simulink model "six_dof_simulation"  (R2020a)
settings: Solver=ode15s  StartTime=0.0  StopTime=1000  FixedStep=0.02  RelTol=1e-3
values from neighbouring files (symbols this model uses):
  u1max = 25*pi/180    (= 0.436332312999)    [initialise.m]
  u1min = -25*pi/180    (= -0.436332312999)    [initialise.m]
  u2max = 10*pi/180    (= 0.174532925199)    [initialise.m]
  u2min = -25*pi/180    (= -0.436332312999)    [initialise.m]
  u3max = 30*pi/180    (= 0.523598775598)    [initialise.m]
  u3min = -30*pi/180    (= -0.523598775598)    [initialise.m]
  u4max = 10*pi/180    (= 0.174532925199)    [initialise.m]
  u4min = 0    [initialise.m]
  u5max = 10*pi/180    (= 0.174532925199)    [initialise.m]
  u5min = 0    [initialise.m]
  x0 = [85 ... (first row only)    [initialise.m]
undefined symbols (not defined in the file or in its folder): RB211, RCAM_plant
libraries: simulink_extras x3, aerolibutil x2, aerolibfltsims x2, aerolibanimutils x1, vrlib x1
settings Model: Creator=Khojasteh Mirza  LastModifiedBy=Khojasteh Mirza
settings SolverCC: InitialStep=0.01
settings DataIOCC: ReturnWorkspaceOutputs=off

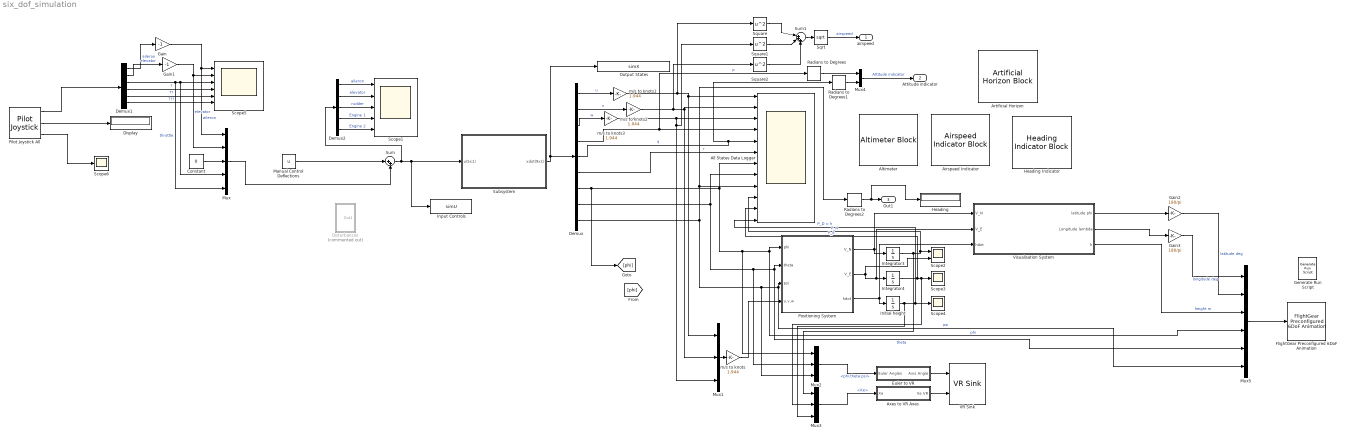
== system six_dof_simulation ==
  Airspeed Indicator : AirspeedIndicatorBlock  ScaleMax=350
  All States Data Logger : Scope  NumInputPorts=12
  Altimeter : AltimeterBlock
  Artificial Horizon : ArtificialHorizonBlock
  Axes to VR Axes : Subsystem
  Constant : Constant  Value=0
  Demux : Demux  Outputs=9
  Demux1 : Demux  Outputs=6
  Demux2 : Demux  Outputs=5
  Display : Display
  Disturbances : Subsystem  Commented=on
  Euler to VR : Subsystem
  FlightGear Preconfigured 6DoF Animation : aerolibfltsims/FlightGear Preconfigured 6DoF Animation  xFlightGearVersion=v2018.1  DestinationIpAddress=127.0.0.1  DestinationPort=5502  SampleTime=1/30  packetVersion=24
  Gain : Gain  Gain=-1
  Gain1 : Gain  Gain=-1
  Gain2 : Gain  Gain=180/pi
  Gain3 : Gain  Gain=180/pi
  Generate Run Script : aerolibfltsims/Generate Run Script  Architecture=Win64  dataFlow=Send  GeometryModelName=757-200-RB211  AirportId=PHNL  RunwayId=26L  InitialAltitude=1000  InitialHeading=260  OffsetDistance=0  OffsetAzimuth=0  InstallScenery=off  DisableShaders=on  OriginAddress=127.0.0.1  DestinationPort=5502  OriginPort=5505  LocalAddress=127.0.0.1  OutputFileName=runfg.bat  FlightGearBaseDirectory=D:\FlightGear 2018.1.1
  Heading : Display
  Heading Indicator : HeadingIndicatorBlock
  Initial height : Integrator  InitialCondition=1000
  Input Controls : ToWorkspace  VariableName=simU  SaveFormat=Timeseries  SampleTime=-1
  Integrator3 : Integrator
  Integrator4 : Integrator
  Manual Control Deflections : Constant  Value=u
  Mux : Mux  Inputs=5
  Mux1 : Mux  Inputs=3
  Mux2 : Mux  Inputs=3
  Mux3 : Mux  Inputs=3
  Mux4 : Mux  Inputs=2
  Mux5 : Mux  Inputs=6
  Output States : ToWorkspace  VariableName=simX  SaveFormat=Timeseries  SampleTime=-1
  Pilot Joystick All : aerolibanimutils/Pilot Joystick  JoystickID=Joystick1  OutputConfiguration=AllOutputs  SampleTime=1/50
  Positioning System : Subsystem
  Radians to Degrees : simulink_extras/Transformations/Radians to Degrees
  Radians to Degrees1 : simulink_extras/Transformations/Radians to Degrees
  Radians to Degrees2 : simulink_extras/Transformations/Radians to Degrees
  Scope1 : Scope  NumInputPorts=5
  Scope2 : Scope  NumInputPorts=2
  Scope3 : Scope
  Scope4 : Scope
  Scope5 : Scope  NumInputPorts=6
  Scope6 : Scope
  Sqrt : Sqrt  SaturateOnIntegerOverflow=on
  Square : Math  Operator=square  SaturateOnIntegerOverflow=on
  Square1 : Math  Operator=square  SaturateOnIntegerOverflow=on
  Square2 : Math  Operator=square  SaturateOnIntegerOverflow=on
  Subsystem : Subsystem
  Sum : Sum  Inputs=|++
  Sum1 : Sum  Inputs=|+++
  VR Sink : vrlib/VR Sink  InstantiateOnLoad=on  SampleTime=0.1  ViewEnable=on  RemoteChange=off  RemoteView=off  FieldsWritten=HL20.rotation.4.1.1.double#HL20.translation.3.1.1.double  WorldFileName=aeroblk_HL20.wrl  WorldDescription=aeroblk_HL20  AutoView=on  VideoDimensions=[]  AllowVariableSize=off
  Visualisation System : Subsystem
  m/s to knots{,1..3} (4 alike) : Gain  Gain=1.944
  airspeed : Outport
  Attitude indicator : Outport  Port=2
  Out1 : Outport  Port=3
  wires:
  Manual Control Deflections/1 -> Sum/1
  Sum/1 -> Demux2/1, Input Controls/1, Subsystem/1(u(5x1))
  Subsystem/1(xdot(9x1)) -> Demux/1, Output States/1
  Demux/4 -> Radians to Degrees/1, All States Data Logger/4  "p"
  Demux/3 -> m/s to knots3/1  "w"
  Demux/2 -> m/s to knots2/1  "v"
  Demux/1 -> m/s to knots1/1  "u"
  Demux/7 -> [phi], All States Data Logger/7, Mux2/1, Mux5/4, Positioning System/1(phi)  "phi"
  Demux/8 -> All States Data Logger/8, Mux2/2, Mux5/5, Positioning System/2(theta)  "theta"
  Demux/9 -> All States Data Logger/9, Radians to Degrees2/1, Mux2/3, Mux5/6, Positioning System/3(psi)  "psi"
  Demux2/1 -> Scope1/1  "aileron"
  Demux2/2 -> Scope1/2  "elevator"
  Demux2/3 -> Scope1/3  "rudder"
  Demux2/4 -> Scope1/4  "Engine 1"
  Demux2/5 -> Scope1/5  "Engine 2"
  Demux/6 -> All States Data Logger/6  "r"
  Positioning System/1(V_N) -> Integrator3/1, Visualisation System/1(V_N)
  Integrator3/1 -> Mux3/1, All States Data Logger/10, Scope2/1  "P_N"
  Positioning System/2(V_E) -> Visualisation System/2(V_E), Integrator4/1, Scope2/2
  Integrator4/1 -> All States Data Logger/11, Mux3/2, Scope3/1  "P_E"
  Initial height/1 -> Mux3/3, All States Data Logger/12, Scope4/1  "P_D = h"
  Positioning System/3(hdot) -> Initial height/1, Visualisation System/3(hdot)
  Axes to VR Axes/1(Xe VR) -> VR Sink/2
  Euler to VR/1(Axis Angle) -> VR Sink/1
  Mux3/1 -> Axes to VR Axes/1(Xe)  "<Xe>"
  Mux2/1 -> Euler to VR/1(Euler Angles)  "<phi;theta;psi>"
  Demux1/4 -> Scope5/4  "?"
  Demux1/1 -> Gain/1  "aileron"
  Demux1/6 -> Scope5/6  "???"
  Pilot Joystick All/1 -> Demux1/1
  Demux1/5 -> Scope5/5  "??"
  Pilot Joystick All/2 -> Display/1
  Demux1/3 -> Mux/5, Scope5/3, Mux/4  "throttle"
  Demux1/2 -> Gain1/1  "elevator"
  Pilot Joystick All/3 -> Scope6/1
  Constant/1 -> Mux/3
  Square/1 -> Sum1/1
  Square1/1 -> Sum1/2
  Square2/1 -> Sum1/3
  Sum1/1 -> Sqrt/1
  Sqrt/1 -> airspeed/1  "airspeed"
  Mux4/1 -> Attitude indicator/1  "Attitude indicator"
  Radians to Degrees/1 -> Mux4/1
  Radians to Degrees1/1 -> Mux4/2
  Radians to Degrees2/1 -> Heading/1, Out1/1
  Gain/1 -> Mux/1, Scope5/1  "aileron"
  Gain1/1 -> Mux/2, Scope5/2  "elevator"
  Mux5/1 -> FlightGear Preconfigured 6DoF Animation/1
  Mux/1 -> Sum/2
  Gain3/1 -> Mux5/1  "longitude deg"
  Gain2/1 -> Mux5/2  "latitude deg"
  Visualisation System/3(h) -> Mux5/3  "height m"
  Visualisation System/1(latitude phi) -> Gain2/1
  Visualisation System/2(Longitude lambda) -> Gain3/1
  Mux1/1 -> m/s to knots/1
  m/s to knots/1 -> Positioning System/4(u,v,w)
  Demux/5 -> All States Data Logger/5, Radians to Degrees1/1  "q"
  m/s to knots1/1 -> Square/1, Mux1/1, All States Data Logger/1
  m/s to knots2/1 -> Square2/1, Mux1/2, All States Data Logger/2
  m/s to knots3/1 -> Square1/1, Mux1/3, All States Data Logger/3

== system six_dof_simulation/Axes to VR Axes ==
  Xe : Inport
  Concatenate : Concatenate  NumInputs=3
  Demux : Demux  Outputs=3
      settings: DisplayOption=none
  rad-->deg : Gain  Gain=-1  SaturateOnIntegerOverflow=on  OutDataTypeStr=Inherit: Same as input  ParamDataTypeStr=Inherit: Same as input
  rad-->deg1 : Gain  Gain=-1  SaturateOnIntegerOverflow=on  OutDataTypeStr=Inherit: Same as input  ParamDataTypeStr=Inherit: Same as input
  Xe VR : Outport  VectorParamsAs1DForOutWhenUnconnected=off
  wires:
  Xe/1 -> Demux/1
  Demux/1 -> Concatenate/1
  Demux/2 -> rad-->deg/1
  Demux/3 -> rad-->deg1/1
  Concatenate/1 -> Xe VR/1
  rad-->deg1/1 -> Concatenate/2
  rad-->deg/1 -> Concatenate/3

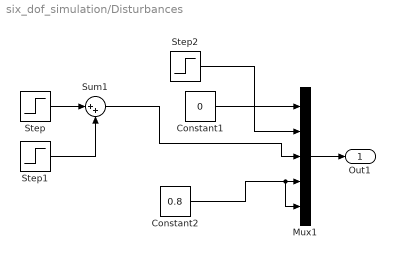
== system six_dof_simulation/Disturbances ==
  Constant1 : Constant  Value=0
  Constant2 : Constant  Value=0.8
  Mux1 : Mux  Inputs=5
  Step : Step  Time=10  After=-25*(pi/180)  SampleTime=0
  Step1 : Step  Time=60  After=10*(pi/180)  SampleTime=0
  Step2 : Step  Time=5  After=-10*(pi/180)  SampleTime=0
  Sum1 : Sum  Inputs=|++
  Out1 : Outport
  wires:
  Mux1/1 -> Out1/1
  Step/1 -> Sum1/1
  Step1/1 -> Sum1/2
  Constant1/1 -> Mux1/1
  Sum1/1 -> Mux1/3
  Step2/1 -> Mux1/2
  Constant2/1 -> Mux1/5, Mux1/4

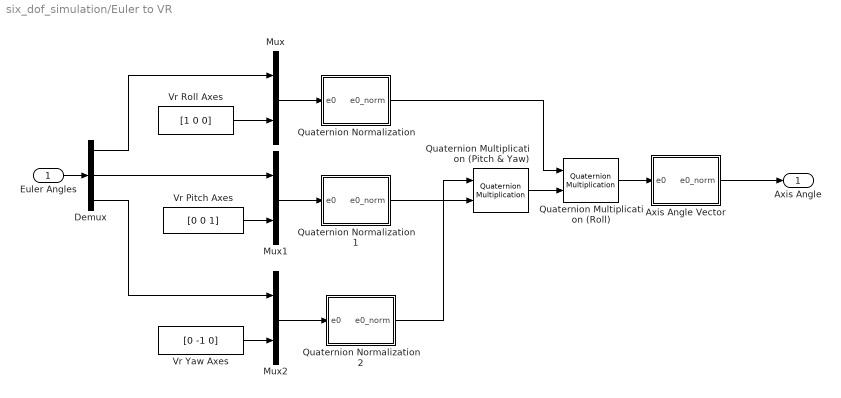
== system six_dof_simulation/Euler to VR ==
  Euler Angles : Inport
  Axis Angle Vector : Subsystem
  Demux : Demux  Outputs=3
      settings: DisplayOption=none
  Mux : Mux  Inputs=2
  Mux1 : Mux  Inputs=2
  Mux2 : Mux  Inputs=2
  Quaternion Multiplication (Pitch & Yaw) : aerolibutil/Quaternion Multiplication
  Quaternion Multiplication (Roll) : aerolibutil/Quaternion Multiplication
  Quaternion Normalization : Subsystem
  Quaternion Normalization1 : Subsystem
  Quaternion Normalization2 : Subsystem
  Vr Pitch Axes : Constant  Value=[0 0 1]
  Vr Roll Axes : Constant  Value=[1 0 0]
  Vr Yaw Axes : Constant  Value=[0 -1 0]
  Axis Angle : Outport  VectorParamsAs1DForOutWhenUnconnected=off
  wires:
  Quaternion Multiplication (Roll)/1 -> Axis Angle Vector/1(e0)
  Quaternion Multiplication (Pitch & Yaw)/1 -> Quaternion Multiplication (Roll)/2
  Axis Angle Vector/1(e0_norm) -> Axis Angle/1
  Quaternion Normalization/1(e0_norm) -> Quaternion Multiplication (Roll)/1
  Quaternion Normalization2/1(e0_norm) -> Quaternion Multiplication (Pitch & Yaw)/1
  Quaternion Normalization1/1(e0_norm) -> Quaternion Multiplication (Pitch & Yaw)/2
  Mux2/1 -> Quaternion Normalization2/1(e0)
  Mux1/1 -> Quaternion Normalization1/1(e0)
  Mux/1 -> Quaternion Normalization/1(e0)
  Demux/3 -> Mux2/1
  Vr Yaw Axes/1 -> Mux2/2
  Demux/2 -> Mux1/1
  Vr Pitch Axes/1 -> Mux1/2
  Demux/1 -> Mux/1
  Vr Roll Axes/1 -> Mux/2
  Euler Angles/1 -> Demux/1

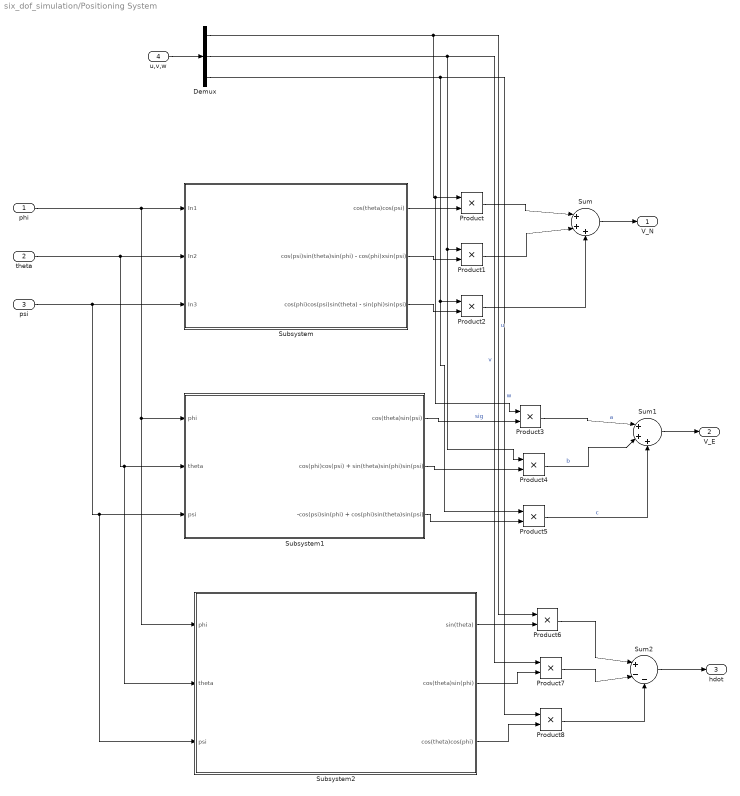
== system six_dof_simulation/Positioning System ==
  phi : Inport
  theta : Inport  Port=2
  psi : Inport  Port=3
  u,v,w : Inport  Port=4
  Demux : Demux  Outputs=3
  Product{,1..8} (9 alike) : Product
  Subsystem : Subsystem
  Subsystem1 : Subsystem
  Subsystem2 : Subsystem
  Sum : Sum  Inputs=|+++
  Sum1 : Sum  Inputs=|+++
  Sum2 : Sum  Inputs=|+--
  V_N : Outport
  V_E : Outport  Port=2
  hdot : Outport  Port=3
  wires:
  u,v,w/1 -> Demux/1
  Demux/1 -> Product6/1, Product3/1, Product/1  "u"
  Demux/2 -> Product7/1, Product4/1, Product1/1  "v"
  Demux/3 -> Product8/1, Product5/1, Product2/1  "w"
  phi/1 -> Subsystem2/1(phi), Subsystem1/1(phi), Subsystem/1(In1)
  psi/1 -> Subsystem/3(In3), Subsystem2/3(psi), Subsystem1/3(psi)
  Subsystem/1(cos(theta)cos(psi)) -> Product/2
  Product/1 -> Sum/1
  Subsystem/2(cos(psi)sin(theta)sin(phi) - cos(phi)xsin(psi)) -> Product1/2
  Product1/1 -> Sum/2
  Subsystem/3(cos(phi)cos(psi)sin(theta) - sin(phi)sin(psi)) -> Product2/2
  Product2/1 -> Sum/3
  Sum/1 -> V_N/1
  theta/1 -> Subsystem2/2(theta), Subsystem1/2(theta), Subsystem/2(In2)
  Sum1/1 -> V_E/1
  Product5/1 -> Sum1/3  "c"
  Product4/1 -> Sum1/2  "b"
  Product3/1 -> Sum1/1  "a"
  Subsystem1/1(cos(theta)sin(psi)) -> Product3/2  "sig"
  Subsystem1/2(cos(phi)cos(psi) + sin(theta)sin(phi)sin(psi)) -> Product4/2
  Subsystem1/3(-cos(psi)sin(phi) + cos(phi)sin(theta)sin(psi)) -> Product5/2
  Subsystem2/1(sin(theta)) -> Product6/2
  Subsystem2/2(cos(theta)sin(phi)) -> Product7/2
  Subsystem2/3(cos(theta)cos(phi)) -> Product8/2
  Product6/1 -> Sum2/1
  Product7/1 -> Sum2/2
  Product8/1 -> Sum2/3
  Sum2/1 -> hdot/1

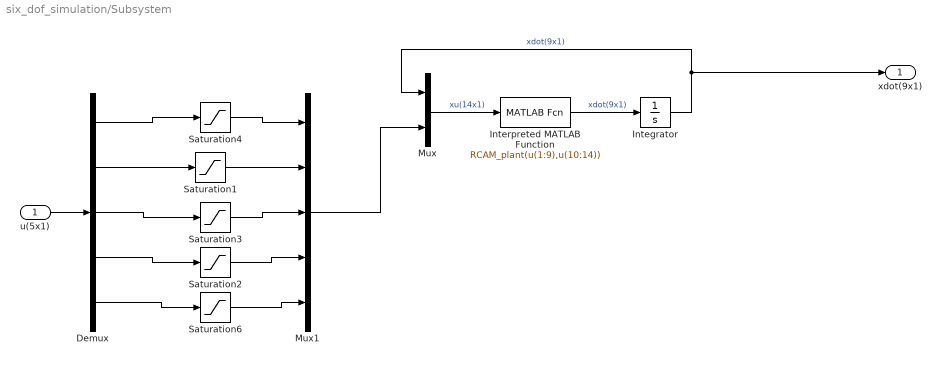
== system six_dof_simulation/Subsystem ==
  u(5x1) : Inport
  Demux : Demux  Outputs=5
  Integrator : Integrator  InitialCondition=x0
  Interpreted MATLAB Function : MATLABFcn  MATLABFcn=RCAM_plant(u(1:9),u(10:14))
  Mux : Mux  Inputs=2
  Mux1 : Mux  Inputs=5
  Saturation1 : Saturate  UpperLimit=u2max  LowerLimit=u2min
  Saturation2 : Saturate  UpperLimit=u4max  LowerLimit=u4min
  Saturation3 : Saturate  UpperLimit=u3max  LowerLimit=u3min
  Saturation4 : Saturate  UpperLimit=u1max  LowerLimit=u1min
  Saturation6 : Saturate  UpperLimit=u5max  LowerLimit=u5min
  xdot(9x1) : Outport
  wires:
  Interpreted MATLAB Function/1 -> Integrator/1  "xdot(9x1)"
  Integrator/1 -> xdot(9x1)/1, Mux/1  "xdot(9x1)"
  Mux/1 -> Interpreted MATLAB Function/1  "xu(14x1)"
  Demux/1 -> Saturation4/1
  Demux/2 -> Saturation1/1
  Demux/3 -> Saturation3/1
  Demux/4 -> Saturation2/1
  Demux/5 -> Saturation6/1
  Saturation4/1 -> Mux1/1
  Saturation1/1 -> Mux1/2
  Saturation3/1 -> Mux1/3
  Saturation2/1 -> Mux1/4
  Saturation6/1 -> Mux1/5
  u(5x1)/1 -> Demux/1
  Mux1/1 -> Mux/2

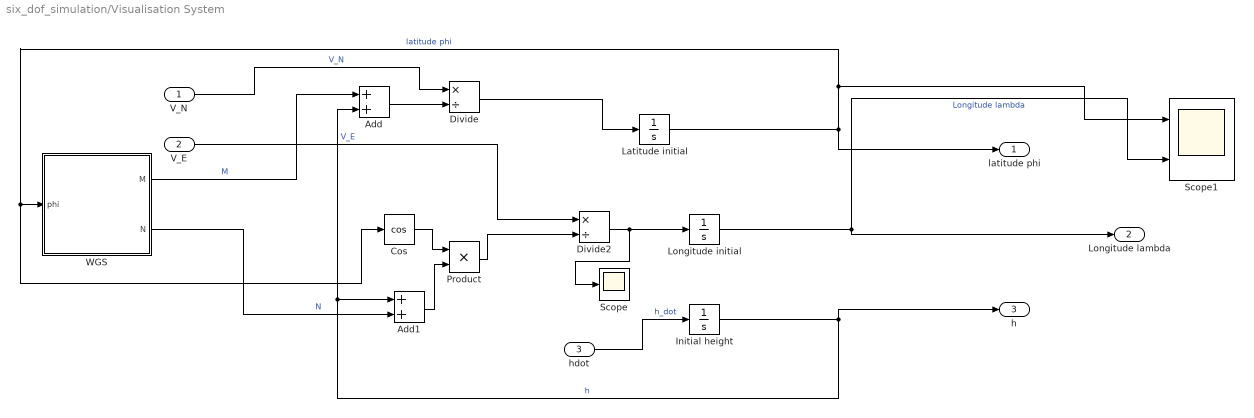
== system six_dof_simulation/Visualisation System ==
  V_N : Inport
  V_E : Inport  Port=2
  hdot : Inport  Port=3
  Add : Sum
  Add1 : Sum
  Cos : Trigonometry  Operator=cos  ApproximationMethod=CORDIC
  Divide : Product  Inputs=*/
  Divide2 : Product  Inputs=*/
  Initial height : Integrator  InitialCondition=1000
  "Latitude initial " : Integrator  InitialCondition=deg2rad(21.32451389)
  Longitude initial : Integrator  InitialCondition=deg2rad(-157.92507222)
  Product : Product
  Scope : Scope
  Scope1 : Scope  NumInputPorts=2
  WGS : Subsystem
  latitude phi : Outport
  Longitude lambda : Outport  Port=2
  h : Outport  Port=3
  wires:
  V_N/1 -> Divide/1  "V_N"
  V_E/1 -> Divide2/1  "V_E"
  WGS/1(M) -> Add/1  "M"
  WGS/2(N) -> Add1/2  "N"
  "Latitude initial "/1 -> latitude phi/1, Cos/1, WGS/1(phi), Scope1/1  "latitude phi"
  Divide/1 -> "Latitude initial "/1
  Initial height/1 -> h/1, Add1/1, Add/2  "h"
  hdot/1 -> Initial height/1  "h_dot"
  Add/1 -> Divide/2
  Longitude initial/1 -> Longitude lambda/1, Scope1/2  "Longitude lambda"
  Add1/1 -> Product/2
  Cos/1 -> Product/1
  Divide2/1 -> Longitude initial/1, Scope/1
  Product/1 -> Divide2/2

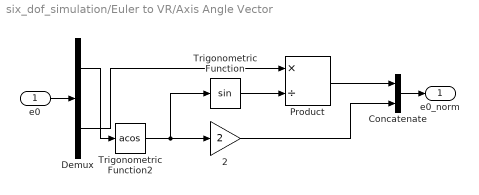
== system six_dof_simulation/Euler to VR/Axis Angle Vector ==
  e0 : Inport
  2 : Gain  Gain=2  SaturateOnIntegerOverflow=on  OutDataTypeStr=Inherit: Same as input  ParamDataTypeStr=Inherit: Same as input
  Concatenate : Concatenate
  Demux : Demux  Outputs=[1 3 ]
      settings: DisplayOption=none
  Product : Product  Inputs=*/  InputSameDT=on  SaturateOnIntegerOverflow=on  OutDataTypeStr=Inherit: Same as first input
  Trigonometric Function : Trigonometry
  Trigonometric Function2 : Trigonometry  Operator=acos
  e0_norm : Outport  VectorParamsAs1DForOutWhenUnconnected=off
  wires:
  Demux/1 -> Trigonometric Function2/1
  Demux/2 -> Product/1
  Concatenate/1 -> e0_norm/1
  Product/1 -> Concatenate/1
  2/1 -> Concatenate/2
  Trigonometric Function/1 -> Product/2
  Trigonometric Function2/1 -> Trigonometric Function/1, 2/1
  e0/1 -> Demux/1

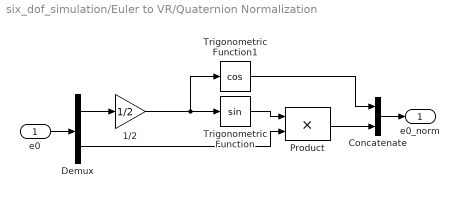
== system six_dof_simulation/Euler to VR/Quaternion Normalization ==
  e0 : Inport
  1/2 : Gain  Gain=1/2  SaturateOnIntegerOverflow=on  OutDataTypeStr=Inherit: Same as input  ParamDataTypeStr=Inherit: Same as input
  Concatenate : Concatenate
  Demux : Demux  Outputs=[1 3]
      settings: DisplayOption=none
  Product : Product  InputSameDT=on  SaturateOnIntegerOverflow=on  OutDataTypeStr=Inherit: Same as first input
  Trigonometric Function : Trigonometry
  Trigonometric Function1 : Trigonometry  Operator=cos
  e0_norm : Outport  VectorParamsAs1DForOutWhenUnconnected=off
  wires:
  Trigonometric Function1/1 -> Concatenate/1
  Demux/2 -> Product/2
  Demux/1 -> 1/2/1
  Concatenate/1 -> e0_norm/1
  Product/1 -> Concatenate/2
  Trigonometric Function/1 -> Product/1
  1/2/1 -> Trigonometric Function1/1, Trigonometric Function/1
  e0/1 -> Demux/1

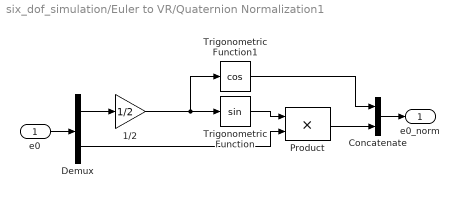
== system six_dof_simulation/Euler to VR/Quaternion Normalization1 ==
  e0 : Inport
  1/2 : Gain  Gain=1/2  SaturateOnIntegerOverflow=on  OutDataTypeStr=Inherit: Same as input  ParamDataTypeStr=Inherit: Same as input
  Concatenate : Concatenate
  Demux : Demux  Outputs=[1 3]
      settings: DisplayOption=none
  Product : Product  InputSameDT=on  SaturateOnIntegerOverflow=on  OutDataTypeStr=Inherit: Same as first input
  Trigonometric Function : Trigonometry
  Trigonometric Function1 : Trigonometry  Operator=cos
  e0_norm : Outport  VectorParamsAs1DForOutWhenUnconnected=off
  wires:
  e0/1 -> Demux/1
  1/2/1 -> Trigonometric Function/1, Trigonometric Function1/1
  Trigonometric Function/1 -> Product/1
  Product/1 -> Concatenate/2
  Concatenate/1 -> e0_norm/1
  Demux/1 -> 1/2/1
  Demux/2 -> Product/2
  Trigonometric Function1/1 -> Concatenate/1

== system six_dof_simulation/Euler to VR/Quaternion Normalization2 ==
  e0 : Inport
  1/2 : Gain  Gain=1/2  SaturateOnIntegerOverflow=on  OutDataTypeStr=Inherit: Same as input  ParamDataTypeStr=Inherit: Same as input
  Concatenate : Concatenate
  Demux : Demux  Outputs=[1 3]
      settings: DisplayOption=none
  Product : Product  InputSameDT=on  SaturateOnIntegerOverflow=on  OutDataTypeStr=Inherit: Same as first input
  Trigonometric Function : Trigonometry
  Trigonometric Function1 : Trigonometry  Operator=cos
  e0_norm : Outport  VectorParamsAs1DForOutWhenUnconnected=off
  wires:
  Trigonometric Function1/1 -> Concatenate/1
  Demux/2 -> Product/2
  Demux/1 -> 1/2/1
  Concatenate/1 -> e0_norm/1
  Product/1 -> Concatenate/2
  Trigonometric Function/1 -> Product/1
  1/2/1 -> Trigonometric Function1/1, Trigonometric Function/1
  e0/1 -> Demux/1

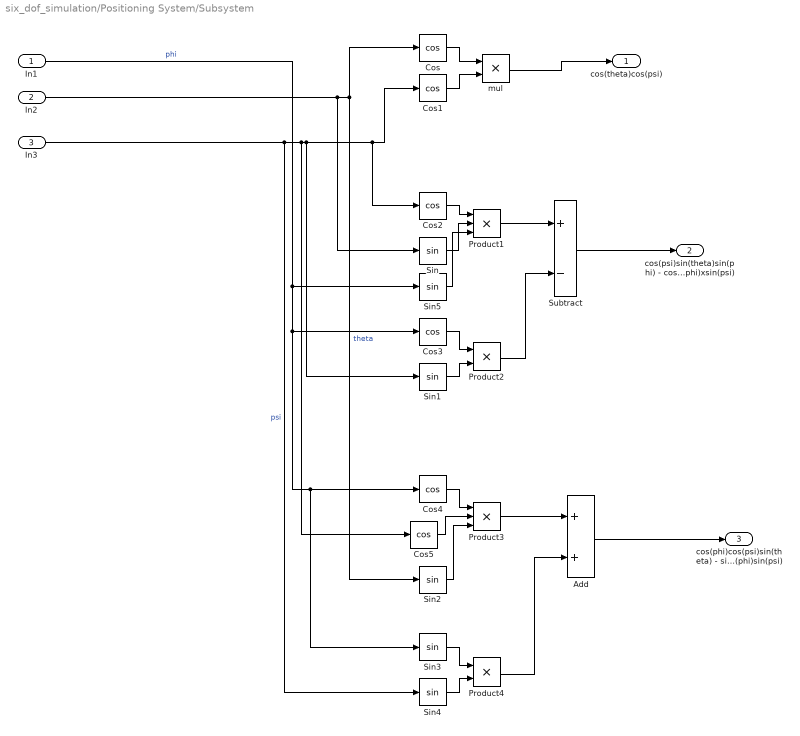
== system six_dof_simulation/Positioning System/Subsystem ==
  In1 : Inport
  In2 : Inport  Port=2
  In3 : Inport  Port=3
  Add : Sum
  Cos{,1..5} (6 alike) : Trigonometry  Operator=cos
  Product1 : Product  Inputs=3
  Product2 : Product
  Product3 : Product  Inputs=3
  Product4 : Product
  Sin{,1..5} (6 alike) : Trigonometry
  Subtract : Sum  Inputs=+-
  mul : Product
  cos(theta)cos(psi) : Outport
  cos(psi)sin(theta)sin(phi) - cos(phi)xsin(psi) : Outport  Port=2
  cos(phi)cos(psi)sin(theta) - sin(phi)sin(psi) : Outport  Port=3
  wires:
  Sin2/1 -> Product3/3
  In1/1 -> Sin3/1, Cos4/1, Cos3/1, Sin5/1  "phi"
  Cos4/1 -> Product3/1
  In2/1 -> Sin/1, Sin2/1, Cos/1  "theta"
  Product3/1 -> Add/1
  Add/1 -> cos(phi)cos(psi)sin(theta) - sin(phi)sin(psi)/1
  Cos5/1 -> Product3/2
  Sin/1 -> Product1/2
  In3/1 -> Sin4/1, Cos5/1, Sin1/1, Cos2/1, Cos1/1  "psi"
  Product1/1 -> Subtract/1
  Subtract/1 -> cos(psi)sin(theta)sin(phi) - cos(phi)xsin(psi)/1
  Cos/1 -> mul/1
  Sin3/1 -> Product4/1
  Product4/1 -> Add/2
  Cos1/1 -> mul/2
  Cos3/1 -> Product2/1
  Cos2/1 -> Product1/1
  Sin4/1 -> Product4/2
  Product2/1 -> Subtract/2
  Sin1/1 -> Product2/2
  mul/1 -> cos(theta)cos(psi)/1
  Sin5/1 -> Product1/3

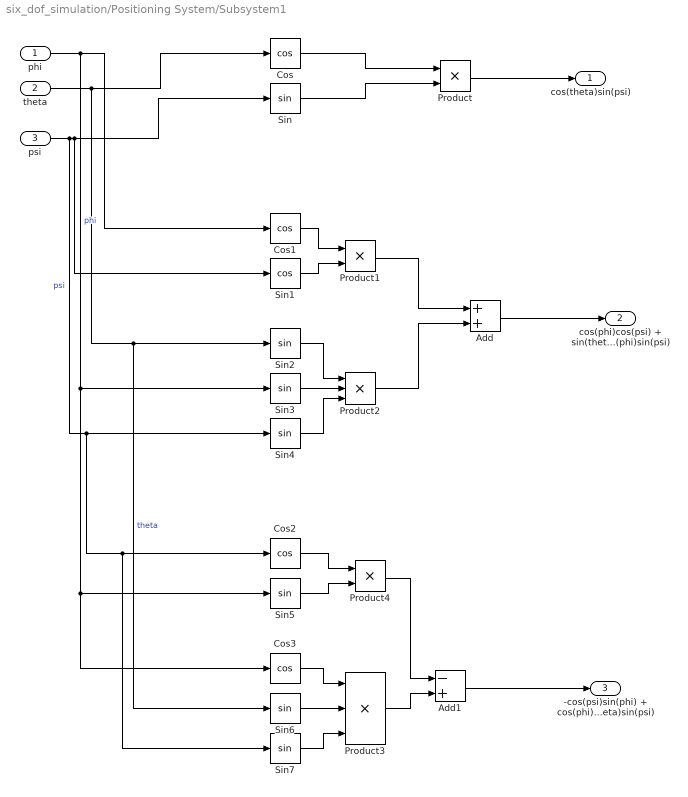
== system six_dof_simulation/Positioning System/Subsystem1 ==
  phi : Inport
  theta : Inport  Port=2
  psi : Inport  Port=3
  Add : Sum
  Add1 : Sum  Inputs=-+
  Cos{,1..3} (4 alike) : Trigonometry  Operator=cos
  Product : Product
  Product1 : Product
  Product2 : Product  Inputs=3
  Product3 : Product  Inputs=3
  Product4 : Product
  Sin{,2..7} (7 alike) : Trigonometry
  Sin1 : Trigonometry  Operator=cos
  cos(theta)sin(psi) : Outport
  cos(phi)cos(psi) + sin(theta)sin(phi)sin(psi) : Outport  Port=2
  -cos(psi)sin(phi) + cos(phi)sin(theta)sin(psi) : Outport  Port=3
  wires:
  theta/1 -> Sin6/1, Sin2/1, Cos/1  "theta"
  psi/1 -> Sin7/1, Cos2/1, Sin4/1, Sin1/1, Sin/1  "psi"
  Cos/1 -> Product/1
  Sin/1 -> Product/2
  phi/1 -> Cos3/1, Sin5/1, Sin3/1, Cos1/1  "phi"
  Sin2/1 -> Product2/1
  Sin3/1 -> Product2/2
  Sin4/1 -> Product2/3
  Cos1/1 -> Product1/1
  Sin1/1 -> Product1/2
  Product1/1 -> Add/1
  Product2/1 -> Add/2
  Cos2/1 -> Product4/1
  Sin5/1 -> Product4/2
  Product4/1 -> Add1/1
  Cos3/1 -> Product3/1
  Sin6/1 -> Product3/2
  Sin7/1 -> Product3/3
  Product3/1 -> Add1/2
  Product/1 -> cos(theta)sin(psi)/1
  Add/1 -> cos(phi)cos(psi) + sin(theta)sin(phi)sin(psi)/1
  Add1/1 -> -cos(psi)sin(phi) + cos(phi)sin(theta)sin(psi)/1

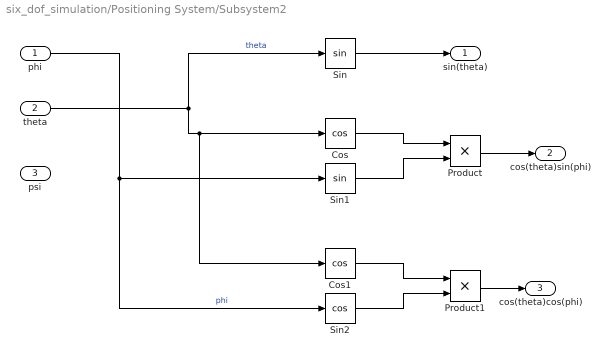
== system six_dof_simulation/Positioning System/Subsystem2 ==
  phi : Inport
  theta : Inport  Port=2
  psi : Inport  Port=3
  Cos : Trigonometry  Operator=cos
  Cos1 : Trigonometry  Operator=cos
  Product : Product
  Product1 : Product
  Sin : Trigonometry
  Sin1 : Trigonometry
  Sin2 : Trigonometry  Operator=cos
  sin(theta) : Outport
  cos(theta)sin(phi) : Outport  Port=2
  cos(theta)cos(phi) : Outport  Port=3
  wires:
  theta/1 -> Cos1/1, Cos/1, Sin/1  "theta"
  Sin/1 -> sin(theta)/1
  phi/1 -> Sin2/1, Sin1/1  "phi"
  Cos/1 -> Product/1
  Sin1/1 -> Product/2
  Cos1/1 -> Product1/1
  Sin2/1 -> Product1/2
  Product/1 -> cos(theta)sin(phi)/1
  Product1/1 -> cos(theta)cos(phi)/1

== system six_dof_simulation/Visualisation System/WGS ==
  phi : Inport
  Constant : Constant  Value=6378137
  Constant1 : Constant  Value=0.081819190842622
  Fcn : Fcn  Expr=u(1)*(1-(u(2)^2))/((1-(u(2)^2)*(sin(u(3))^2))^(3/2))
  Fcn1 : Fcn  Expr=u(1)/sqrt(1-u(2)^2)*(sin(u(3))^2)
  Mux : Mux  Inputs=3
  M : Outport
  N : Outport  Port=2
  wires:
  Constant/1 -> Mux/1
  Constant1/1 -> Mux/2
  phi/1 -> Mux/3
  Mux/1 -> Fcn1/1, Fcn/1
  Fcn1/1 -> N/1
  Fcn/1 -> M/1
